simulink model "sim_LAB4"  (R2025b)
settings: Solver=VariableStepAuto  StartTime=0.0  StopTime=100  FixedStep=0.001  RelTol=1e-3
values from neighbouring files (symbols this model uses):
  C = Ts/(Tc+Ts)    [CM_LAB4.m]
  C12 = -(body.m*body.zb+2*mot.rot.m*mot.rot.zb)*wheel.r    [CM_LAB4.m]
  Fv = F + ((2*gbox.N^2*mot.Kt*mot.Ke)/(mot.R))*[1 -1;-1 1]    [CM_LAB4.m]
  G2 = -(body.m*body.zb+2*mot.rot.m*mot.rot.zb)*g    [CM_LAB4.m]
  K = dlqr(Phi, Gamma, Q, R)    [CM_LAB4.m]
  K_e = dlqr(Phi_e,Gamma_e,Q_e,R)    [CM_LAB4.m]
  M11 = 2*wheel.Iyy + 2*gbox.N^2*mot.rot.Iyy+(body.m+2*wheel.m+2*mot.rot.m)*wheel.r^2    [CM_LAB4.m]
  M21_1 = 2*gbox.N*(1-gbox.N)*mot.rot.Iyy    [CM_LAB4.m]
  M21_2 = (body.m*body.zb+2*mot.rot.m*mot.rot.zb)*wheel.r    [CM_LAB4.m]
  M22 = body.Iyy+2*(1-gbox.N)^2*mot.rot.Iyy+body.m*(body.zb^2)+2*mot.rot.m*(mot.rot.zb^2)    [CM_LAB4.m]
  Nu = N(5)    [CM_LAB4.m]
  Nx = N(1:4)    [CM_LAB4.m]
  Tc = 1/(2*pi*fc)    (= 0.497359197162)    [CM_LAB4.m]
undefined symbols (not defined in the file or in its folder): DiscIntNeverNeededParam, drv, g, gbox, mot, ms22g, sens, Ts, wheel, x0
settings Model: Creator=Gioele  LastModifiedBy=Gioele

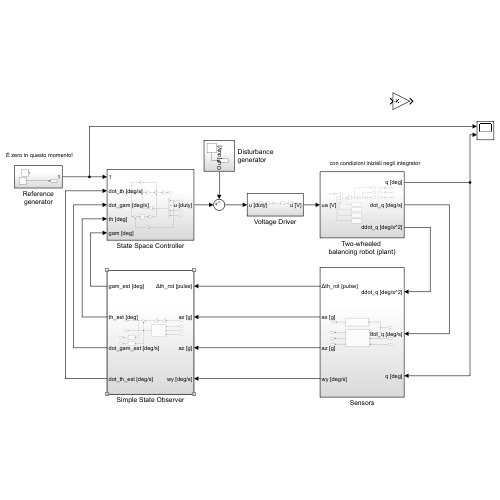
[thumbnail: Simulink's stored preview of the top-level diagram]
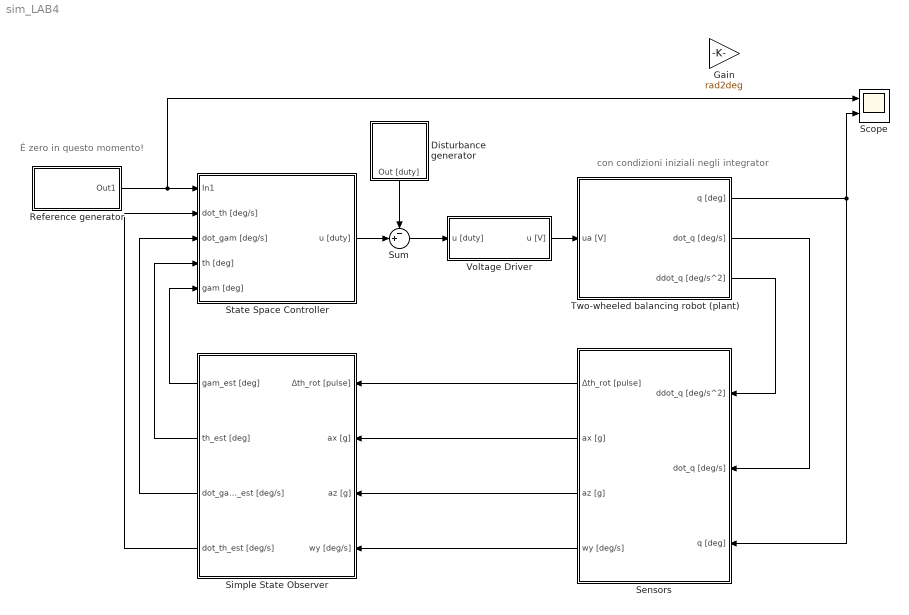
== system sim_LAB4 ==
  note: con condizioni iniziali negli integrator
  note: É zero in questo momento!
  Disturbance generator : Subsystem
  Gain : Gain  Gain=rad2deg
  Reference generator : Subsystem
  Scope : Scope  NumInputPorts=2
      settings: ActiveDisplayYMinimum=-33.168501609758138  ActiveDisplayYMaximum=177.93421302068316
  Sensors : Subsystem
  Simple State Observer : Subsystem
  State Space Controller : Subsystem
  Sum : Sum  Inputs=-+|
  Two-wheeled balancing robot (plant) : Subsystem
  Voltage Driver : Subsystem
  wires:
  Two-wheeled balancing robot (plant)/1(q [deg]) -> Scope/2, Sensors/3(q [deg])
  Two-wheeled balancing robot (plant)/2(dot_q [deg/s]) -> Sensors/2(dot_q [deg/s])
  Two-wheeled balancing robot (plant)/3(ddot_q [deg/s^2]) -> Sensors/1(ddot_q [deg/s^2])
  Sensors/1(Δth_rot [pulse]) -> Simple State Observer/1(Δth_rot [pulse])
  Sensors/2(ax [g]) -> Simple State Observer/2(ax [g])
  Sensors/3(az [g]) -> Simple State Observer/3(az [g])
  Sensors/4(wy [deg/s]) -> Simple State Observer/4(wy [deg/s])
  Simple State Observer/1(gam_est [deg]) -> State Space Controller/5(gam [deg])
  Simple State Observer/2(th_est [deg]) -> State Space Controller/4(th [deg])
  Simple State Observer/3(dot_gam_est [deg/s]) -> State Space Controller/3(dot_gam [deg/s])
  Simple State Observer/4(dot_th_est [deg/s]) -> State Space Controller/2(dot_th [deg/s])
  Sum/1 -> Voltage Driver/1(u [duty])
  Disturbance generator/1(Out [duty]) -> Sum/1
  State Space Controller/1(u [duty]) -> Sum/2
  Voltage Driver/1(u [V]) -> Two-wheeled balancing robot (plant)/1(ua [V])
  Reference generator/1(Out1) -> Scope/1, State Space Controller/1(In1)

== system sim_LAB4/Disturbance generator ==
  Constant : Constant  Value=0  SampleTime=Ts
  Out [duty] : Outport
  wires:
  Constant/1 -> Out [duty]/1

== system sim_LAB4/Reference generator ==
  Constant : Constant  Value=0  SampleTime=Ts
  Step : Step  Time=0  After=0.1/wheel.r  SampleTime=Ts
  Out1 : Outport
  wires:
  Constant/1 -> Out1/1

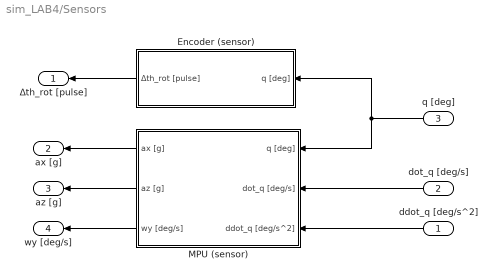
== system sim_LAB4/Sensors ==
  ddot_q [deg/s^2] : Inport
  dot_q [deg/s] : Inport  Port=2
  q [deg] : Inport  Port=3
  Encoder (sensor) : Subsystem
  MPU (sensor) : Subsystem
  Δth_rot [pulse] : Outport
  ax [g] : Outport  Port=2
  az [g] : Outport  Port=3
  wy [deg/s] : Outport  Port=4
  wires:
  MPU (sensor)/1(ax [g]) -> ax [g]/1
  MPU (sensor)/3(wy [deg/s]) -> wy [deg/s]/1
  q [deg]/1 -> Encoder (sensor)/1(q [deg]), MPU (sensor)/1(q [deg])
  ddot_q [deg/s^2]/1 -> MPU (sensor)/3(ddot_q [deg/s^2])
  Encoder (sensor)/1(Δth_rot [pulse]) -> Δth_rot [pulse]/1
  dot_q [deg/s]/1 -> MPU (sensor)/2(dot_q [deg/s])
  MPU (sensor)/2(az [g]) -> az [g]/1

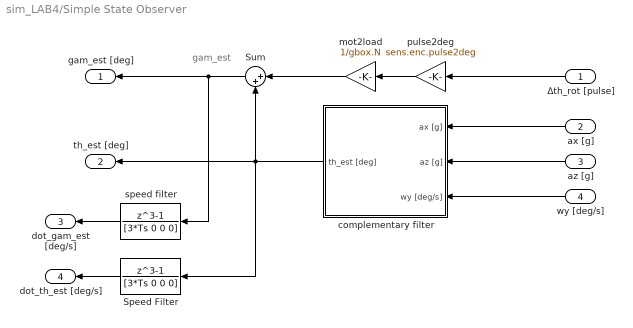
== system sim_LAB4/Simple State Observer ==
  note: gam_est
  Δth_rot [pulse] : Inport
  ax [g] : Inport  Port=2
  az [g] : Inport  Port=3
  wy [deg/s] : Inport  Port=4
  Speed Filter : DiscreteTransferFcn  Numerator=[1 0 0 -1]  Denominator=[3*Ts 0 0 0]
  Sum : Sum  Inputs=|++
  complementary filter : Subsystem
  mot2load : Gain  Gain=1/gbox.N
  pulse2deg : Gain  Gain=sens.enc.pulse2deg
  speed filter : DiscreteTransferFcn  Numerator=[1 0 0 -1]  Denominator=[3*Ts 0 0 0]
  gam_est [deg] : Outport
  th_est [deg] : Outport  Port=2
  dot_gam_est [deg/s] : Outport  Port=3
  dot_th_est [deg/s] : Outport  Port=4
  wires:
  mot2load/1 -> Sum/1
  Speed Filter/1 -> dot_th_est [deg/s]/1
  complementary filter/1(th_est [deg]) -> Speed Filter/1, th_est [deg]/1, Sum/2
  az [g]/1 -> complementary filter/2(az [g])
  speed filter/1 -> dot_gam_est [deg/s]/1
  pulse2deg/1 -> mot2load/1
  Δth_rot [pulse]/1 -> pulse2deg/1
  wy [deg/s]/1 -> complementary filter/3(wy [deg/s])
  Sum/1 -> gam_est [deg]/1, speed filter/1
  ax [g]/1 -> complementary filter/1(ax [g])

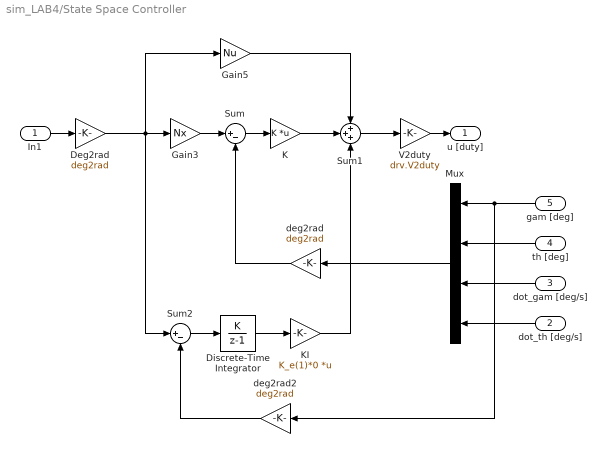
== system sim_LAB4/State Space Controller ==
  In1 : Inport
  dot_th [deg/s] : Inport  Port=2
  dot_gam [deg/s] : Inport  Port=3
  th [deg] : Inport  Port=4
  gam [deg] : Inport  Port=5
  Deg2rad : Gain  Gain=deg2rad
  Discrete-Time Integrator : DiscreteIntegrator  IntegratorMethod=Accumulation: Forward Euler  SampleTime=Ts  ICPrevOutput=DiscIntNeverNeededParam  ICPrevScaledInput=DiscIntNeverNeededParam
  Gain3 : Gain  Gain=Nx
  Gain5 : Gain  Gain=Nu
  K : Gain  Gain=K  Multiplication=Matrix(K*u)
  KI : Gain  Gain=K_e(1)*0  Multiplication=Matrix(K*u)
  Mux : Mux
  Sum : Sum  Inputs=|+-
  Sum1 : Sum  Inputs=+++
  Sum2 : Sum  Inputs=|+-
  V2duty : Gain  Gain=drv.V2duty
  deg2rad : Gain  Gain=deg2rad
  deg2rad2 : Gain  Gain=deg2rad
  u [duty] : Outport
  wires:
  K/1 -> Sum1/2
  deg2rad/1 -> Sum/2
  Gain3/1 -> Sum/1
  Mux/1 -> deg2rad/1
  Sum1/1 -> V2duty/1
  Sum/1 -> K/1
  Gain5/1 -> Sum1/1
  V2duty/1 -> u [duty]/1
  KI/1 -> Sum1/3
  Sum2/1 -> Discrete-Time Integrator/1
  Discrete-Time Integrator/1 -> KI/1
  deg2rad2/1 -> Sum2/2
  In1/1 -> Deg2rad/1
  gam [deg]/1 -> Mux/1, deg2rad2/1
  th [deg]/1 -> Mux/2
  dot_gam [deg/s]/1 -> Mux/3
  dot_th [deg/s]/1 -> Mux/4
  Deg2rad/1 -> Sum2/1, Gain5/1, Gain3/1

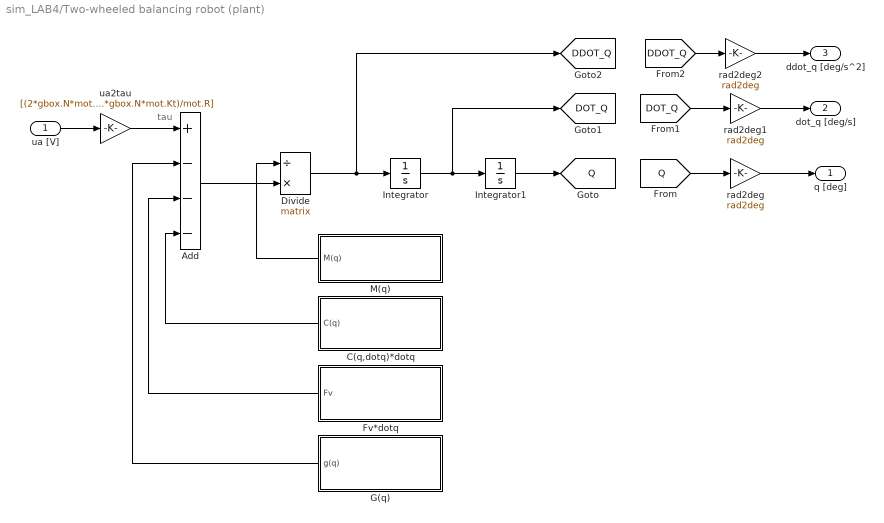
== system sim_LAB4/Two-wheeled balancing robot (plant) ==
  note: tau
  ua [V] : Inport
  Add : Sum  Inputs=+---
  C(q,dotq)*dotq : Subsystem
  Divide : Product  Inputs=/*  Multiplication=Matrix(*)
  Fv*dotq : Subsystem
  G(q) : Subsystem
  Integrator : Integrator  InitialCondition=[ x0(3);x0(4)]
  Integrator1 : Integrator  InitialCondition=[x0(1); x0(2)]
  M(q) : Subsystem
  rad2deg : Gain  Gain=rad2deg
  rad2deg1 : Gain  Gain=rad2deg
  rad2deg2 : Gain  Gain=rad2deg
  ua2tau : Gain  Gain=[(2*gbox.N*mot.Kt)/mot.R , -(2*gbox.N*mot.Kt)/mot.R]
  q [deg] : Outport
  dot_q [deg/s] : Outport  Port=2
  ddot_q [deg/s^2] : Outport  Port=3
  tag scope: DDOT_Q=global, DOT_Q=global, Q=global
  wires:
  ua2tau/1 -> Add/1
  Divide/1 -> [DDOT_Q], Integrator/1
  ua [V]/1 -> ua2tau/1
  [DOT_Q] -> rad2deg1/1
  Integrator/1 -> [DOT_Q], Integrator1/1
  Add/1 -> Divide/2
  Integrator1/1 -> [Q]
  rad2deg/1 -> q [deg]/1
  [Q] -> rad2deg/1
  [DDOT_Q] -> rad2deg2/1
  rad2deg2/1 -> ddot_q [deg/s^2]/1
  M(q)/1(M(q)) -> Divide/1
  rad2deg1/1 -> dot_q [deg/s]/1
  Fv*dotq/1(Fv) -> Add/3
  G(q)/1(g(q)) -> Add/2
  C(q,dotq)*dotq/1(C(q)) -> Add/4

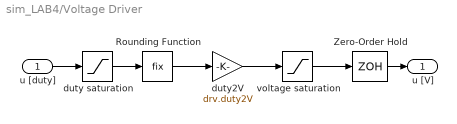
== system sim_LAB4/Voltage Driver ==
  u [duty] : Inport
  Rounding Function : Rounding  Operator=fix
  Zero-Order Hold : ZeroOrderHold  SampleTime=Ts
  duty saturation : Saturate  UpperLimit=drv.dutymax  LowerLimit=-drv.dutymax
  duty2V : Gain  Gain=drv.duty2V
  voltage saturation : Saturate  UpperLimit=drv.Vbus  LowerLimit=-drv.Vbus
  u [V] : Outport
  wires:
  Rounding Function/1 -> duty2V/1
  duty2V/1 -> voltage saturation/1
  duty saturation/1 -> Rounding Function/1
  Zero-Order Hold/1 -> u [V]/1
  voltage saturation/1 -> Zero-Order Hold/1
  u [duty]/1 -> duty saturation/1

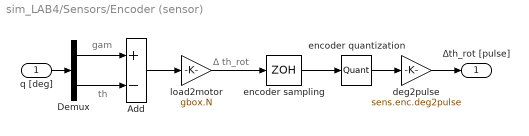
== system sim_LAB4/Sensors/Encoder (sensor) ==
  note: Δ th_rot
  note: th
  note: gam
  q [deg] : Inport
  Add : Sum  Inputs=+-
  Demux : Demux  Outputs=2
  deg2pulse : Gain  Gain=sens.enc.deg2pulse
  encoder quantization : Quantizer  QuantizationInterval=sens.enc.pulse2deg
  encoder sampling : ZeroOrderHold  SampleTime=Ts
  load2motor : Gain  Gain=gbox.N
  Δth_rot [pulse] : Outport
  wires:
  encoder quantization/1 -> deg2pulse/1
  encoder sampling/1 -> encoder quantization/1
  load2motor/1 -> encoder sampling/1
  Demux/2 -> Add/2
  deg2pulse/1 -> Δth_rot [pulse]/1
  Demux/1 -> Add/1
  q [deg]/1 -> Demux/1
  Add/1 -> load2motor/1

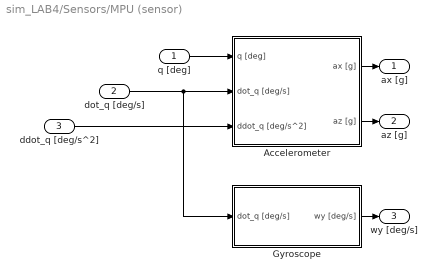
== system sim_LAB4/Sensors/MPU (sensor) ==
  q [deg] : Inport
  dot_q [deg/s] : Inport  Port=2
  ddot_q [deg/s^2] : Inport  Port=3
  Accelerometer : Subsystem
  Gyroscope : Subsystem
  ax [g] : Outport
  az [g] : Outport  Port=2
  wy [deg/s] : Outport  Port=3
  wires:
  dot_q [deg/s]/1 -> Gyroscope/1(dot_q [deg/s]), Accelerometer/2(dot_q [deg/s])
  ddot_q [deg/s^2]/1 -> Accelerometer/3(ddot_q [deg/s^2])
  q [deg]/1 -> Accelerometer/1(q [deg])
  Gyroscope/1(wy [deg/s]) -> wy [deg/s]/1
  Accelerometer/2(az [g]) -> az [g]/1
  Accelerometer/1(ax [g]) -> ax [g]/1

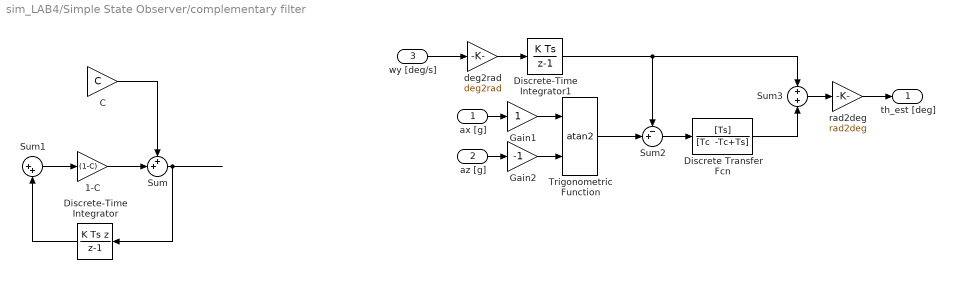
== system sim_LAB4/Simple State Observer/complementary filter ==
  ax [g] : Inport
  az [g] : Inport  Port=2
  wy [deg/s] : Inport  Port=3
  1-C : Gain  Gain=(1-C)
  C : Gain  Gain=C
  Discrete Transfer Fcn : DiscreteTransferFcn  Numerator=[Ts]  Denominator="[Tc  -Tc+Ts]"
  Discrete-Time Integrator : DiscreteIntegrator  IntegratorMethod=Integration: Backward Euler  gainval=1  SampleTime=Ts  ICPrevOutput=DiscIntNeverNeededParam  ICPrevScaledInput=DiscIntNeverNeededParam
  Discrete-Time Integrator1 : DiscreteIntegrator  SampleTime=Ts  ICPrevOutput=DiscIntNeverNeededParam  ICPrevScaledInput=DiscIntNeverNeededParam
  Gain1 : Gain
  Gain2 : Gain  Gain=-1
  Sum : Sum  Inputs=++|
  Sum1 : Sum  Inputs=|++
  Sum2 : Sum  Inputs=-+|
  Sum3 : Sum  Inputs=+|+
  Trigonometric Function : Trigonometry  Operator=atan2
  deg2rad : Gain  Gain=deg2rad
  rad2deg : Gain  Gain=rad2deg
  th_est [deg] : Outport
  wires:
  Gain2/1 -> Trigonometric Function/2
  Gain1/1 -> Trigonometric Function/1
  wy [deg/s]/1 -> deg2rad/1
  az [g]/1 -> Gain2/1
  ax [g]/1 -> Gain1/1
  rad2deg/1 -> th_est [deg]/1
  Sum3/1 -> rad2deg/1
  ? -> C/1
  C/1 -> Sum/1
  1-C/1 -> Sum/2
  Discrete-Time Integrator/1 -> Sum1/2
  Sum/1 -> Discrete-Time Integrator/1
  Sum1/1 -> 1-C/1
  Trigonometric Function/1 -> Sum2/2
  Discrete Transfer Fcn/1 -> Sum3/2
  Sum2/1 -> Discrete Transfer Fcn/1
  deg2rad/1 -> Discrete-Time Integrator1/1
  Discrete-Time Integrator1/1 -> Sum2/1, Sum3/1

== system sim_LAB4/Two-wheeled balancing robot (plant)/C(q,dotq)*dotq ==
  Matrix C(q,dot_q) : Subsystem
  Product1 : Product  Multiplication=Matrix(*)
  C(q) : Outport
  wires:
  [Q] -> Matrix C(q,dot_q)/1(q)
  Matrix C(q,dot_q)/1(C(q,dot_q)) -> Product1/1
  [DOT_Q] -> Product1/2
  Product1/1 -> C(q)/1
  [DOT_Q] -> Matrix C(q,dot_q)/2(dot_q)

== system sim_LAB4/Two-wheeled balancing robot (plant)/Fv*dotq ==
  Constant - Fv1 : Constant  Value=Fv  SampleTime=Ts
  Product2 : Product  Multiplication=Matrix(*)
  Fv : Outport
  wires:
  Constant - Fv1/1 -> Product2/1
  [DOT_Q] -> Product2/2
  Product2/1 -> Fv/1

== system sim_LAB4/Two-wheeled balancing robot (plant)/G(q) ==
  Matrix g(q) : Subsystem
  g(q) : Outport
  wires:
  [Q] -> Matrix g(q)/1(q)
  Matrix g(q)/1(g(q)) -> g(q)/1

== system sim_LAB4/Two-wheeled balancing robot (plant)/M(q) ==
  Matrix M(q) : Subsystem
  M(q) : Outport
  wires:
  [Q] -> Matrix M(q)/1(q)
  Matrix M(q)/1(M(q)) -> M(q)/1

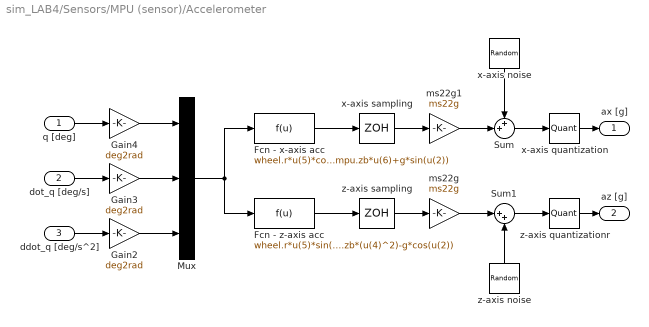
== system sim_LAB4/Sensors/MPU (sensor)/Accelerometer ==
  q [deg] : Inport
  dot_q [deg/s] : Inport  Port=2
  ddot_q [deg/s^2] : Inport  Port=3
  Fcn - x-axis acc : Fcn  Expr=wheel.r*u(5)*cos(u(2))+sens.mpu.zb*u(6)+g*sin(u(2))
  Fcn - z-axis acc : Fcn  Expr=wheel.r*u(5)*sin(u(2))-sens.mpu.zb*(u(4)^2)-g*cos(u(2))
  Gain2 : Gain  Gain=deg2rad
  Gain3 : Gain  Gain=deg2rad
  Gain4 : Gain  Gain=deg2rad
  Mux : Mux  Inputs=3
  Sum : Sum  Inputs=++|
  Sum1 : Sum  Inputs=|++
  ms22g : Gain  Gain=ms22g
  ms22g1 : Gain  Gain=ms22g
  x-axis quantization : Quantizer  QuantizationInterval=sens.mpu.acc.LSB2g
  x-axis sampling : ZeroOrderHold  SampleTime=Ts
  x-axis noise : RandomNumber  Variance=sens.mpu.acc.noisevar  SampleTime=Ts
  z-axis sampling : ZeroOrderHold  SampleTime=Ts
  z-axis quantizationr : Quantizer  QuantizationInterval=sens.mpu.acc.LSB2g
  z-axis noise : RandomNumber  Variance=sens.mpu.acc.noisevar  SampleTime=Ts
  ax [g] : Outport
  az [g] : Outport  Port=2
  wires:
  x-axis noise/1 -> Sum/1
  Sum1/1 -> z-axis quantizationr/1
  x-axis sampling/1 -> ms22g1/1
  Mux/1 -> Fcn - z-axis acc/1, Fcn - x-axis acc/1
  Gain2/1 -> Mux/3
  Sum/1 -> x-axis quantization/1
  x-axis quantization/1 -> ax [g]/1
  z-axis sampling/1 -> ms22g/1
  ms22g1/1 -> Sum/2
  Gain4/1 -> Mux/1
  z-axis noise/1 -> Sum1/2
  ms22g/1 -> Sum1/1
  Fcn - x-axis acc/1 -> x-axis sampling/1
  Fcn - z-axis acc/1 -> z-axis sampling/1
  Gain3/1 -> Mux/2
  dot_q [deg/s]/1 -> Gain3/1
  z-axis quantizationr/1 -> az [g]/1
  ddot_q [deg/s^2]/1 -> Gain2/1
  q [deg]/1 -> Gain4/1

== system sim_LAB4/Sensors/MPU (sensor)/Gyroscope ==
  dot_q [deg/s] : Inport
  Selector : Selector  InputPortWidth=2  IndexOptions=Index vector (dialog)  Indices=[2]  OutputSizes=1
  Sum2 : Sum  Inputs=++|
  y-axis quantization : Quantizer  QuantizationInterval=sens.mpu.gyro.LSB2degs
  y-axis sampling : ZeroOrderHold  SampleTime=Ts
  y-axis noise : RandomNumber  Variance=sens.mpu.gyro.noisevar  SampleTime=Ts
  wy [deg/s] : Outport
  wires:
  Selector/1 -> y-axis sampling/1
  y-axis noise/1 -> Sum2/1
  dot_q [deg/s]/1 -> Selector/1
  Sum2/1 -> y-axis quantization/1
  y-axis sampling/1 -> Sum2/2
  y-axis quantization/1 -> wy [deg/s]/1

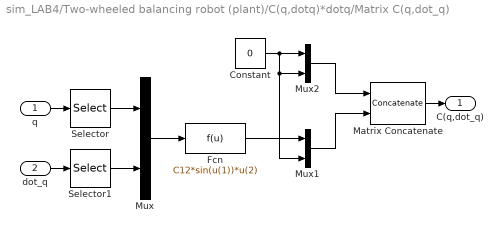
== system sim_LAB4/Two-wheeled balancing robot (plant)/C(q,dotq)*dotq/Matrix C(q,dot_q) ==
  q : Inport
  dot_q : Inport  Port=2
  Constant : Constant  Value=0  SampleTime=Ts
  Fcn : Fcn  Expr=C12*sin(u(1))*u(2)
  Matrix Concatenate : Concatenate  Mode=Multidimensional array  ConcatenateDimension=2
  Mux : Mux  Inputs=2
  Mux1 : Mux  Inputs=2
  Mux2 : Mux  Inputs=2
  Selector : Selector  InputPortWidth=2  IndexOptions=Index vector (dialog)  Indices=[2]  OutputSizes=1
  Selector1 : Selector  InputPortWidth=2  IndexOptions=Index vector (dialog)  Indices=[2]  OutputSizes=1
  C(q,dot_q) : Outport
  wires:
  Selector1/1 -> Mux/2
  Mux/1 -> Fcn/1
  Constant/1 -> Mux2/2, Mux1/2, Mux2/1
  Mux2/1 -> Matrix Concatenate/1
  Selector/1 -> Mux/1
  Mux1/1 -> Matrix Concatenate/2
  Fcn/1 -> Mux1/1
  Matrix Concatenate/1 -> C(q,dot_q)/1
  dot_q/1 -> Selector1/1
  q/1 -> Selector/1

== system sim_LAB4/Two-wheeled balancing robot (plant)/G(q)/Matrix g(q) ==
  q : Inport
  Constant - g1 : Constant  Value=0  SampleTime=Ts
  Fcn - g2(q) : Fcn  Expr=G2*sin(u)
  Mux : Mux  Inputs=2
  Selector : Selector  InputPortWidth=2  IndexOptions=Index vector (dialog)  Indices=[2]  OutputSizes=1
  g(q) : Outport
  wires:
  Selector/1 -> Fcn - g2(q)/1
  Constant - g1/1 -> Mux/1
  Mux/1 -> g(q)/1
  Fcn - g2(q)/1 -> Mux/2
  q/1 -> Selector/1

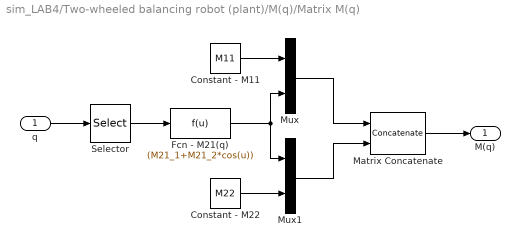
== system sim_LAB4/Two-wheeled balancing robot (plant)/M(q)/Matrix M(q) ==
  q : Inport
  Constant - M11 : Constant  Value=M11  SampleTime=Ts
  Constant - M22 : Constant  Value=M22  SampleTime=Ts
  Fcn - M21(q) : Fcn  Expr=(M21_1+M21_2*cos(u))
  Matrix Concatenate : Concatenate  Mode=Multidimensional array  ConcatenateDimension=2
  Mux : Mux  Inputs=2
  Mux1 : Mux  Inputs=2
  Selector : Selector  InputPortWidth=2  IndexOptions=Index vector (dialog)  Indices=[2]  OutputSizes=1
  M(q) : Outport
  wires:
  Matrix Concatenate/1 -> M(q)/1
  Selector/1 -> Fcn - M21(q)/1
  Fcn - M21(q)/1 -> Mux/2, Mux1/1
  Constant - M11/1 -> Mux/1
  q/1 -> Selector/1
  Constant - M22/1 -> Mux1/2
  Mux1/1 -> Matrix Concatenate/2
  Mux/1 -> Matrix Concatenate/1
